simulink model "flightController"  (Simulink 9.1)
settings: Solver=ode3  StartTime=0  StopTime=TFinal  FixedStep=Ts  RelTol=1e-3  EnableMultiTasking=on
undefined symbols (not defined in the file): Controller, DiscIntNeverNeededParam, g, Ts, Vehicle
libraries: F_Line_block x89
settings Model: LogicAnalyzerSignalOrdering=201c873a-a194-43e1-85c1-7820e482cbc3,e6e4670c-19f9-4e85-8601-519539bde157  Creator=The MathWorks, Inc.  LastModifiedBy=dongw
settings DataIOCC: LimitDataPoints=on
settings OptimizationCC: BlockReduction=off  DefaultParameterBehavior=Inlined  BufferReuse=off  PassReuseOutputArgsThreshold=0  LifeSpan=auto
settings DebuggingCC: AlgebraicLoopMsg=none  UnderspecifiedInitializationDetection=Simplified  MergeDetectMultiDrivingBlocksExec=error  ParameterPrecisionLossMsg=none  ParameterTunabilityLossMsg=error  UnconnectedInputMsg=none  UnconnectedOutputMsg=none  UnconnectedLineMsg=none  BusObjectLabelMismatch=error
settings HardwareCC: ProdLargestAtomicInteger=Long  ProdLargestAtomicFloat=Float  ProdIntDivRoundTo=Zero  ProdEndianess=LittleEndian  ProdHWDeviceType=ARM Compatible->ARM 9
settings ModelReferenceCC: ModelReferenceNumInstancesAllowed=Single
settings RTWCC: GenerateReport=on  LaunchReport=on
settings CodeAppCC: ForceParamTrailComments=on  MaxIdLength=63  OperatorAnnotations=on  MATLABSourceComments=on
settings GRTTargetCC: CombineOutputUpdateFcns=on  GRTInterface=off
settings ConfigComp: CovSFcnEnable=off

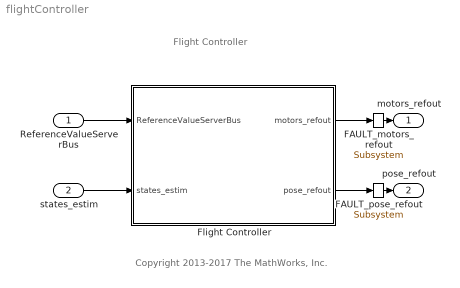
== system flightController ==
  note: Flight Controller
  note: Copyright 2013-2017 The MathWorks, Inc.
  ReferenceValueServerBus : Inport  OutDataTypeStr=Bus: CommandBus  BusOutputAsStruct=on
  states_estim : Inport  Port=2  OutDataTypeStr=Bus: statesEstim_t  BusOutputAsStruct=on
  Flight Controller : Subsystem
  motors_refout : Outport
  FAULT_motors_refout : F_Line_block/Subsystem
  pose_refout : Outport  Port=2
  FAULT_pose_refout : F_Line_block/Subsystem
  wires:
  ReferenceValueServerBus/1 -> Flight Controller/1(ReferenceValueServerBus)
  states_estim/1 -> Flight Controller/2(states_estim)
  Flight Controller/2(pose_refout) -> FAULT_pose_refout/1
  FAULT_pose_refout/1 -> pose_refout/1
  Flight Controller/1(motors_refout) -> FAULT_motors_refout/1
  FAULT_motors_refout/1 -> motors_refout/1

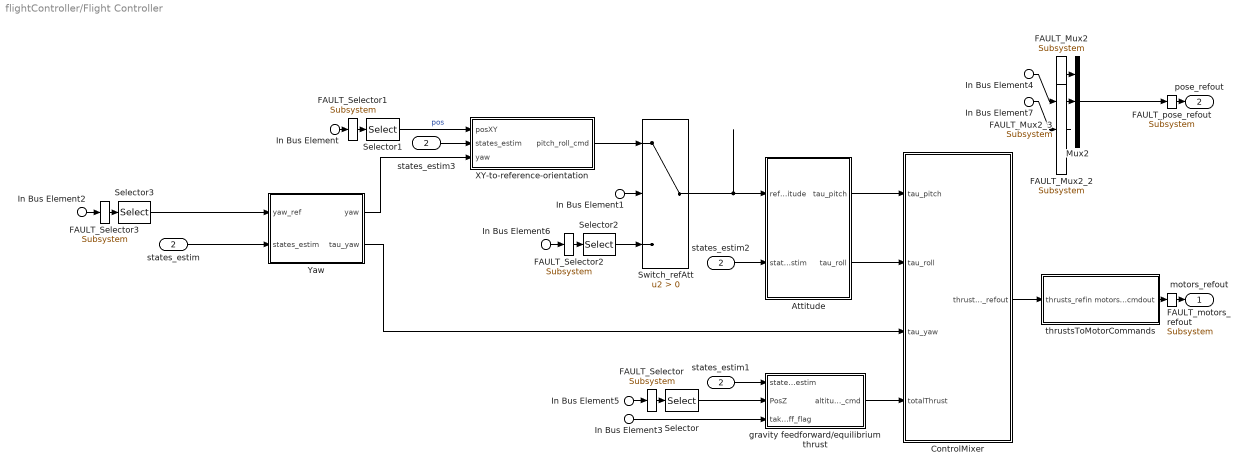
== system flightController/Flight Controller ==
  In Bus Element1 : Inport  PortName=ReferenceValueServerBus  Element=controlModePosVSOrient
  In Bus Element : Inport  PortName=ReferenceValueServerBus  Element=pos_ref
  In Bus Element4 : Inport  PortName=ReferenceValueServerBus  Element=pos_ref
  In Bus Element5 : Inport  PortName=ReferenceValueServerBus  Element=pos_ref
  In Bus Element2 : Inport  PortName=ReferenceValueServerBus  Element=orient_ref
  In Bus Element6 : Inport  PortName=ReferenceValueServerBus  Element=orient_ref
  In Bus Element7 : Inport  PortName=ReferenceValueServerBus  Element=orient_ref
  In Bus Element3 : Inport  PortName=ReferenceValueServerBus  Element=takeoff_flag
  states_estim : Inport  Port=2
  Attitude : Subsystem
  ControlMixer : Subsystem
  Mux2 : Mux  Inputs=3
  FAULT_Mux2 : F_Line_block/Subsystem
  FAULT_Mux2_2 : F_Line_block/Subsystem
  FAULT_Mux2_3 : F_Line_block/Subsystem
  Selector : Selector  InputPortWidth=3  IndexOptions=Index vector (dialog)  Indices=3  OutputSizes=1
  FAULT_Selector{,1..3} (4 alike) : F_Line_block/Subsystem
  Selector1 : Selector  InputPortWidth=3  IndexOptions=Index vector (dialog)  Indices=[1 2]  OutputSizes=1
  Selector2 : Selector  InputPortWidth=3  IndexOptions=Index vector (dialog)  Indices=[2 3]  OutputSizes=1
  Selector3 : Selector  InputPortWidth=3  IndexOptions=Index vector (dialog)  Indices=1  OutputSizes=1
  Switch_refAtt : Switch  Criteria=u2 > Threshold
  XY-to-reference-orientation : Subsystem
  Yaw : Subsystem
  gravity feedforward/equilibrium thrust : Subsystem
  states_estim1 : InportShadow  Port=2
  states_estim2 : InportShadow  Port=2
  states_estim3 : InportShadow  Port=2
  thrustsToMotorCommands : Subsystem
  motors_refout : Outport
  FAULT_motors_refout : F_Line_block/Subsystem
  pose_refout : Outport  Port=2
  FAULT_pose_refout : F_Line_block/Subsystem
  wires:
  thrustsToMotorCommands/1(motors_cmdout) -> FAULT_motors_refout/1
  FAULT_motors_refout/1 -> motors_refout/1
  In Bus Element1/1 -> Switch_refAtt/2
  XY-to-reference-orientation/1(pitch_roll_cmd) -> Switch_refAtt/1
  In Bus Element2/1 -> FAULT_Selector3/1
  FAULT_Selector3/1 -> Selector3/1
  In Bus Element/1 -> FAULT_Selector1/1
  FAULT_Selector1/1 -> Selector1/1
  Selector3/1 -> Yaw/1(yaw_ref)
  Selector1/1 -> XY-to-reference-orientation/1(posXY)  "pos"
  ControlMixer/1(thrusts_refout) -> thrustsToMotorCommands/1(thrusts_refin)
  In Bus Element3/1 -> gravity feedforward/equilibrium thrust/3(takeoff_flag)
  states_estim/1 -> Yaw/2(states_estim)
  Switch_refAtt/1 -> Attitude/1(refAttitude)
  ?FAULT_Sum4/1 -> ?Sum4/1
  FAULT_Mux2/1 -> Mux2/1
  Yaw/1(yaw) -> XY-to-reference-orientation/3(yaw)
  gravity feedforward/equilibrium thrust/1(altitude_cmd) -> ControlMixer/4(totalThrust)
  Mux2/1 -> FAULT_pose_refout/1
  FAULT_pose_refout/1 -> pose_refout/1
  Attitude/1(tau_pitch) -> ControlMixer/1(tau_pitch)
  Attitude/2(tau_roll) -> ControlMixer/2(tau_roll)
  Yaw/2(tau_yaw) -> ControlMixer/3(tau_yaw)
  states_estim1/1 -> gravity feedforward/equilibrium thrust/1(states_estim)
  states_estim2/1 -> Attitude/2(states_estim)
  states_estim3/1 -> XY-to-reference-orientation/2(states_estim)
  In Bus Element4/1 -> FAULT_Mux2/1
  FAULT_Mux2/1 -> Mux2/1
  Selector/1 -> gravity feedforward/equilibrium thrust/2(PosZ)
  In Bus Element5/1 -> FAULT_Selector/1
  FAULT_Selector/1 -> Selector/1
  In Bus Element6/1 -> FAULT_Selector2/1
  FAULT_Selector2/1 -> Selector2/1
  Selector2/1 -> Switch_refAtt/3
  In Bus Element7/1 -> FAULT_Mux2_2/1
  FAULT_Mux2_2/1 -> Mux2/2

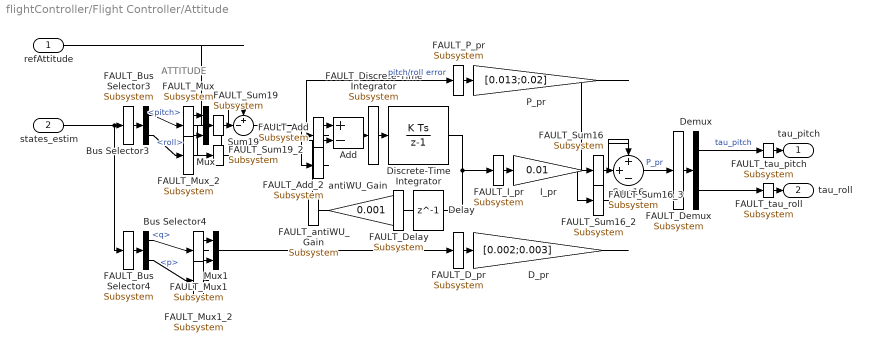
== system flightController/Flight Controller/Attitude ==
  note: ATTITUDE
  refAttitude : Inport
  states_estim : Inport  Port=2
  Add : Sum  Inputs=+-
  FAULT_Add : F_Line_block/Subsystem
  FAULT_Add_2 : F_Line_block/Subsystem
  Bus Selector3 : BusSelector  OutputSignals=pitch,roll
  FAULT_Bus Selector3 : F_Line_block/Subsystem
  Bus Selector4 : BusSelector  OutputSignals=q,p
  FAULT_Bus Selector4 : F_Line_block/Subsystem
  D_pr : Gain  Gain=[0.002;0.003]
  FAULT_D_pr : F_Line_block/Subsystem
  Delay : Delay  DelayLength=1  InitialCondition=0
  FAULT_Delay : F_Line_block/Subsystem
  Demux : Demux  Outputs=2
  FAULT_Demux : F_Line_block/Subsystem
  Discrete-Time Integrator : DiscreteIntegrator  SampleTime=Ts  LimitOutput=on  UpperSaturationLimit=2  LowerSaturationLimit=-2  ICPrevOutput=DiscIntNeverNeededParam  ICPrevScaledInput=DiscIntNeverNeededParam
  FAULT_Discrete-Time Integrator : F_Line_block/Subsystem
  I_pr : Gain  Gain=0.01
  FAULT_I_pr : F_Line_block/Subsystem
  Mux : Mux  Inputs=2
  FAULT_Mux : F_Line_block/Subsystem
  FAULT_Mux_2 : F_Line_block/Subsystem
  Mux1 : Mux  Inputs=2
  FAULT_Mux1 : F_Line_block/Subsystem
  FAULT_Mux1_2 : F_Line_block/Subsystem
  P_pr : Gain  Gain=[0.013;0.02]
  FAULT_P_pr : F_Line_block/Subsystem
  Sum16 : Sum  Inputs=++-  AccumDataTypeStr=single  OutDataTypeStr=single  SaturateOnIntegerOverflow=on
  FAULT_Sum16 : F_Line_block/Subsystem
  FAULT_Sum16_2 : F_Line_block/Subsystem
  FAULT_Sum16_3 : F_Line_block/Subsystem
  Sum19 : Sum  Inputs=+-|
  FAULT_Sum19 : F_Line_block/Subsystem
  FAULT_Sum19_2 : F_Line_block/Subsystem
  antiWU_Gain : Gain  Gain=0.001
  FAULT_antiWU_Gain : F_Line_block/Subsystem
  tau_pitch : Outport
  FAULT_tau_pitch : F_Line_block/Subsystem
  tau_roll : Outport  Port=2
  FAULT_tau_roll : F_Line_block/Subsystem
  wires:
  Sum16/1 -> FAULT_Demux/1  "P_pr"
  FAULT_Demux/1 -> Demux/1
  antiWU_Gain/1 -> FAULT_Add_2/1
  FAULT_Add_2/1 -> Add/2
  Add/1 -> FAULT_Discrete-Time Integrator/1
  FAULT_Discrete-Time Integrator/1 -> Discrete-Time Integrator/1
  Bus Selector3/1 -> FAULT_Mux/1  "<pitch>"
  FAULT_Mux/1 -> Mux/1
  Bus Selector4/1 -> FAULT_Mux1/1  "<q>"
  FAULT_Mux1/1 -> Mux1/1
  P_pr/1 -> FAULT_Sum16/1
  FAULT_Sum16/1 -> Sum16/1
  I_pr/1 -> FAULT_Sum16_2/1
  FAULT_Sum16_2/1 -> Sum16/2
  Sum19/1 -> FAULT_Add/1, FAULT_P_pr/1  "pitch/roll error"
  FAULT_Add/1 -> Add/1
  FAULT_P_pr/1 -> P_pr/1
  Discrete-Time Integrator/1 -> FAULT_Delay/1, FAULT_I_pr/1
  FAULT_Delay/1 -> Delay/1
  FAULT_I_pr/1 -> I_pr/1
  Delay/1 -> FAULT_antiWU_Gain/1
  FAULT_antiWU_Gain/1 -> antiWU_Gain/1
  Demux/1 -> FAULT_tau_pitch/1  "tau_pitch"
  FAULT_tau_pitch/1 -> tau_pitch/1
  Demux/2 -> FAULT_tau_roll/1
  FAULT_tau_roll/1 -> tau_roll/1
  D_pr/1 -> ?
  FAULT_Sum16/1 -> Sum16/1
  states_estim/1 -> FAULT_Bus Selector3/1, FAULT_Bus Selector4/1
  FAULT_Bus Selector3/1 -> Bus Selector3/1
  FAULT_Bus Selector4/1 -> Bus Selector4/1
  refAttitude/1 -> FAULT_Sum19/1
  FAULT_Sum19/1 -> Sum19/1
  Mux/1 -> FAULT_Sum19_2/1
  FAULT_Sum19_2/1 -> Sum19/2
  Bus Selector3/2 -> FAULT_Mux_2/1  "<roll>"
  FAULT_Mux_2/1 -> Mux/2
  Mux1/1 -> FAULT_D_pr/1
  FAULT_D_pr/1 -> D_pr/1
  Bus Selector4/2 -> FAULT_Mux1_2/1  "<p>"
  FAULT_Mux1_2/1 -> Mux1/2

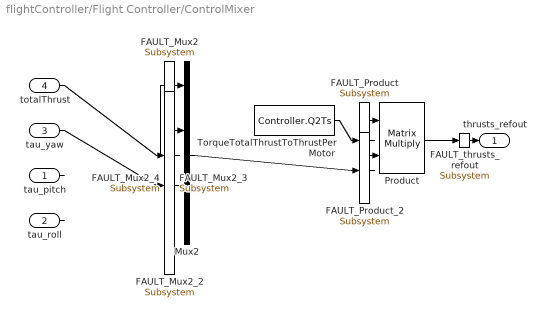
== system flightController/Flight Controller/ControlMixer ==
  tau_pitch : Inport
  tau_roll : Inport  Port=2
  tau_yaw : Inport  Port=3
  totalThrust : Inport  Port=4
  Mux2 : Mux
  FAULT_Mux2 : F_Line_block/Subsystem
  FAULT_Mux2_2 : F_Line_block/Subsystem
  FAULT_Mux2_3 : F_Line_block/Subsystem
  FAULT_Mux2_4 : F_Line_block/Subsystem
  Product : Product  Multiplication=Matrix(*)  RndMeth=Zero
  FAULT_Product : F_Line_block/Subsystem
  FAULT_Product_2 : F_Line_block/Subsystem
  TorqueTotalThrustToThrustPerMotor : Constant  Value=Controller.Q2Ts  OutDataTypeStr=single
  thrusts_refout : Outport
  FAULT_thrusts_refout : F_Line_block/Subsystem
  wires:
  Product/1 -> FAULT_thrusts_refout/1
  FAULT_thrusts_refout/1 -> thrusts_refout/1
  tau_roll/1 -> ?
  FAULT_Mux2/1 -> Mux2/1
  tau_pitch/1 -> ?
  FAULT_Mux2/1 -> Mux2/1
  tau_yaw/1 -> FAULT_Mux2_2/1
  FAULT_Mux2_2/1 -> Mux2/2
  totalThrust/1 -> FAULT_Mux2/1
  FAULT_Mux2/1 -> Mux2/1
  TorqueTotalThrustToThrustPerMotor/1 -> FAULT_Product/1
  FAULT_Product/1 -> Product/1
  Mux2/1 -> FAULT_Product_2/1
  FAULT_Product_2/1 -> Product/2

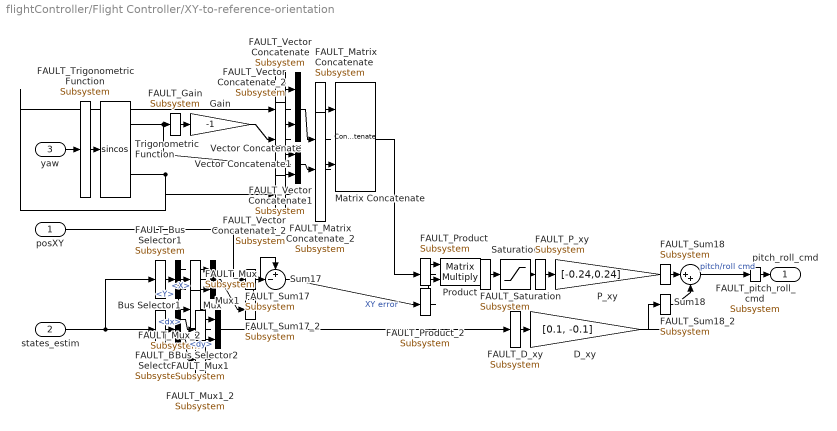
== system flightController/Flight Controller/XY-to-reference-orientation ==
  posXY : Inport
  states_estim : Inport  Port=2
  yaw : Inport  Port=3
  Bus Selector1 : BusSelector  OutputSignals=X,Y
  FAULT_Bus Selector1 : F_Line_block/Subsystem
  Bus Selector2 : BusSelector  OutputSignals=dx,dy
  FAULT_Bus Selector2 : F_Line_block/Subsystem
  D_xy : Gain  Gain=[0.1, -0.1]  ParamDataTypeStr=single  OutDataTypeStr=single  SaturateOnIntegerOverflow=on
  FAULT_D_xy : F_Line_block/Subsystem
  Gain : Gain  Gain=-1
  FAULT_Gain : F_Line_block/Subsystem
  Matrix Concatenate : Concatenate  Mode=Multidimensional array  ConcatenateDimension=2
  FAULT_Matrix Concatenate : F_Line_block/Subsystem
  FAULT_Matrix Concatenate_2 : F_Line_block/Subsystem
  Mux : Mux  Inputs=2
  FAULT_Mux : F_Line_block/Subsystem
  FAULT_Mux_2 : F_Line_block/Subsystem
  Mux1 : Mux  Inputs=2
  FAULT_Mux1 : F_Line_block/Subsystem
  FAULT_Mux1_2 : F_Line_block/Subsystem
  P_xy : Gain  Gain=[-0.24,0.24]  ParamDataTypeStr=single  OutDataTypeStr=single  SaturateOnIntegerOverflow=on
  FAULT_P_xy : F_Line_block/Subsystem
  Product : Product  Multiplication=Matrix(*)  OutDataTypeStr=single  RndMeth=Zero
  FAULT_Product : F_Line_block/Subsystem
  FAULT_Product_2 : F_Line_block/Subsystem
  Saturation : Saturate  UpperLimit=3  LowerLimit=-3  OutDataTypeStr=single
  FAULT_Saturation : F_Line_block/Subsystem
  Sum17 : Sum  Inputs=+-|  AccumDataTypeStr=single
  FAULT_Sum17 : F_Line_block/Subsystem
  FAULT_Sum17_2 : F_Line_block/Subsystem
  Sum18 : Sum  Inputs=|++  AccumDataTypeStr=single  OutDataTypeStr=single  SaturateOnIntegerOverflow=on
  FAULT_Sum18 : F_Line_block/Subsystem
  FAULT_Sum18_2 : F_Line_block/Subsystem
  Trigonometric Function : Trigonometry  Operator=sincos
  FAULT_Trigonometric Function : F_Line_block/Subsystem
  Vector Concatenate : Concatenate
  FAULT_Vector Concatenate : F_Line_block/Subsystem
  FAULT_Vector Concatenate_2 : F_Line_block/Subsystem
  Vector Concatenate1 : Concatenate
  FAULT_Vector Concatenate1 : F_Line_block/Subsystem
  FAULT_Vector Concatenate1_2 : F_Line_block/Subsystem
  pitch_roll_cmd : Outport
  FAULT_pitch_roll_cmd : F_Line_block/Subsystem
  wires:
  yaw/1 -> FAULT_Trigonometric Function/1
  FAULT_Trigonometric Function/1 -> Trigonometric Function/1
  Saturation/1 -> FAULT_P_xy/1
  FAULT_P_xy/1 -> P_xy/1
  P_xy/1 -> FAULT_Sum18/1
  FAULT_Sum18/1 -> Sum18/1
  Sum17/1 -> FAULT_Product_2/1  "XY error"
  FAULT_Product_2/1 -> Product/2
  posXY/1 -> FAULT_Sum17/1
  FAULT_Sum17/1 -> Sum17/1
  Bus Selector2/1 -> FAULT_Mux1/1  "<dx>"
  FAULT_Mux1/1 -> Mux1/1
  states_estim/1 -> FAULT_Bus Selector1/1, FAULT_Bus Selector2/1
  FAULT_Bus Selector1/1 -> Bus Selector1/1
  FAULT_Bus Selector2/1 -> Bus Selector2/1
  Sum18/1 -> FAULT_pitch_roll_cmd/1  "pitch/roll cmd"
  FAULT_pitch_roll_cmd/1 -> pitch_roll_cmd/1
  D_xy/1 -> FAULT_Sum18_2/1
  FAULT_Sum18_2/1 -> Sum18/2
  Bus Selector1/1 -> FAULT_Mux/1  "<X>"
  FAULT_Mux/1 -> Mux/1
  Product/1 -> FAULT_Saturation/1
  FAULT_Saturation/1 -> Saturation/1
  Trigonometric Function/1 -> FAULT_Gain/1, FAULT_Vector Concatenate1/1
  FAULT_Gain/1 -> Gain/1
  FAULT_Vector Concatenate1/1 -> Vector Concatenate1/1
  Trigonometric Function/2 -> FAULT_Vector Concatenate1_2/1, FAULT_Vector Concatenate/1
  FAULT_Vector Concatenate1_2/1 -> Vector Concatenate1/2
  FAULT_Vector Concatenate/1 -> Vector Concatenate/1
  Gain/1 -> FAULT_Vector Concatenate_2/1
  FAULT_Vector Concatenate_2/1 -> Vector Concatenate/2
  Vector Concatenate/1 -> FAULT_Matrix Concatenate/1
  FAULT_Matrix Concatenate/1 -> Matrix Concatenate/1
  Vector Concatenate1/1 -> FAULT_Matrix Concatenate_2/1
  FAULT_Matrix Concatenate_2/1 -> Matrix Concatenate/2
  Matrix Concatenate/1 -> FAULT_Product/1
  FAULT_Product/1 -> Product/1
  Bus Selector1/2 -> FAULT_Mux_2/1  "<Y>"
  FAULT_Mux_2/1 -> Mux/2
  Mux/1 -> FAULT_Sum17_2/1
  FAULT_Sum17_2/1 -> Sum17/2
  Mux1/1 -> FAULT_D_xy/1
  FAULT_D_xy/1 -> D_xy/1
  Bus Selector2/2 -> FAULT_Mux1_2/1  "<dy>"
  FAULT_Mux1_2/1 -> Mux1/2

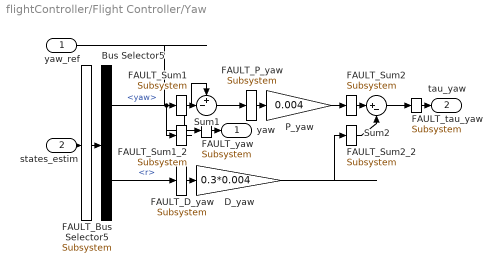
== system flightController/Flight Controller/Yaw ==
  yaw_ref : Inport
  states_estim : Inport  Port=2
  Bus Selector5 : BusSelector  OutputSignals=yaw,r
  FAULT_Bus Selector5 : F_Line_block/Subsystem
  D_yaw : Gain  Gain=0.3*0.004
  FAULT_D_yaw : F_Line_block/Subsystem
  P_yaw : Gain  Gain=0.004  ParamDataTypeStr=single  OutDataTypeStr=single
  FAULT_P_yaw : F_Line_block/Subsystem
  Sum1 : Sum  Inputs=+-|  AccumDataTypeStr=single  OutDataTypeStr=single  SaturateOnIntegerOverflow=on
  FAULT_Sum1 : F_Line_block/Subsystem
  FAULT_Sum1_2 : F_Line_block/Subsystem
  Sum2 : Sum  Inputs=|+-
  FAULT_Sum2 : F_Line_block/Subsystem
  FAULT_Sum2_2 : F_Line_block/Subsystem
  yaw : Outport
  FAULT_yaw : F_Line_block/Subsystem
  tau_yaw : Outport  Port=2
  FAULT_tau_yaw : F_Line_block/Subsystem
  wires:
  D_yaw/1 -> FAULT_Sum2_2/1
  FAULT_Sum2_2/1 -> Sum2/2
  P_yaw/1 -> FAULT_Sum2/1
  FAULT_Sum2/1 -> Sum2/1
  Bus Selector5/2 -> FAULT_D_yaw/1  "<r>"
  FAULT_D_yaw/1 -> D_yaw/1
  Sum1/1 -> FAULT_P_yaw/1
  FAULT_P_yaw/1 -> P_yaw/1
  states_estim/1 -> FAULT_Bus Selector5/1
  FAULT_Bus Selector5/1 -> Bus Selector5/1
  Sum2/1 -> FAULT_tau_yaw/1
  FAULT_tau_yaw/1 -> tau_yaw/1
  Bus Selector5/1 -> FAULT_yaw/1, FAULT_Sum1_2/1  "<yaw>"
  FAULT_yaw/1 -> yaw/1
  FAULT_Sum1_2/1 -> Sum1/2
  yaw_ref/1 -> FAULT_Sum1/1
  FAULT_Sum1/1 -> Sum1/1

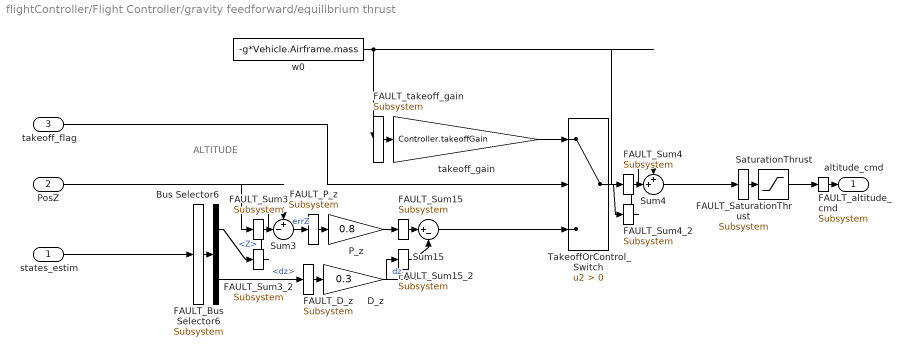
== system flightController/Flight Controller/gravity feedforward/equilibrium thrust ==
  note: ALTITUDE
  states_estim : Inport
  PosZ : Inport  Port=2
  takeoff_flag : Inport  Port=3
  Bus Selector6 : BusSelector  OutputSignals=Z,dz
  FAULT_Bus Selector6 : F_Line_block/Subsystem
  D_z : Gain  Gain=0.3  ParamDataTypeStr=single  OutDataTypeStr=single  SaturateOnIntegerOverflow=on
  FAULT_D_z : F_Line_block/Subsystem
  P_z : Gain  Gain=0.8  ParamDataTypeStr=single  OutDataTypeStr=single  SaturateOnIntegerOverflow=on
  FAULT_P_z : F_Line_block/Subsystem
  SaturationThrust : Saturate  UpperLimit=4*Controller.totalThrustMaxRelative*Controller.motorsThrustPerMotorMax  LowerLimit=-4*Controller.totalThrustMaxRelative*Controller.motorsThrustPerMotorMax  OutDataTypeStr=single
  FAULT_SaturationThrust : F_Line_block/Subsystem
  Sum15 : Sum  Inputs=|+-  AccumDataTypeStr=single  OutDataTypeStr=single  SaturateOnIntegerOverflow=on
  FAULT_Sum15 : F_Line_block/Subsystem
  FAULT_Sum15_2 : F_Line_block/Subsystem
  Sum3 : Sum  Inputs=+-|  AccumDataTypeStr=single  OutDataTypeStr=single  SaturateOnIntegerOverflow=on
  FAULT_Sum3 : F_Line_block/Subsystem
  FAULT_Sum3_2 : F_Line_block/Subsystem
  Sum4 : Sum  Inputs=++|  AccumDataTypeStr=single  OutDataTypeStr=single  SaturateOnIntegerOverflow=on
  FAULT_Sum4 : F_Line_block/Subsystem
  FAULT_Sum4_2 : F_Line_block/Subsystem
  TakeoffOrControl_Switch : Switch  Criteria=u2 > Threshold
  takeoff_gain : Gain  Gain=Controller.takeoffGain  ParamDataTypeStr=single  OutDataTypeStr=single  SaturateOnIntegerOverflow=on
  FAULT_takeoff_gain : F_Line_block/Subsystem
  w0 : Constant  Value=-g*Vehicle.Airframe.mass  OutDataTypeStr=single  SampleTime=Ts
  altitude_cmd : Outport
  FAULT_altitude_cmd : F_Line_block/Subsystem
  wires:
  Sum3/1 -> FAULT_P_z/1  "errZ"
  FAULT_P_z/1 -> P_z/1
  TakeoffOrControl_Switch/1 -> FAULT_Sum4_2/1
  FAULT_Sum4_2/1 -> Sum4/2
  Bus Selector6/1 -> FAULT_Sum3_2/1  "<Z>"
  FAULT_Sum3_2/1 -> Sum3/2
  Bus Selector6/2 -> FAULT_D_z/1  "<dz>"
  FAULT_D_z/1 -> D_z/1
  w0/1 -> FAULT_Sum4/1, FAULT_takeoff_gain/1
  FAULT_Sum4/1 -> Sum4/1
  FAULT_takeoff_gain/1 -> takeoff_gain/1
  D_z/1 -> FAULT_Sum15_2/1  "dz"
  FAULT_Sum15_2/1 -> Sum15/2
  takeoff_gain/1 -> TakeoffOrControl_Switch/1
  takeoff_flag/1 -> TakeoffOrControl_Switch/2
  PosZ/1 -> FAULT_Sum3/1
  FAULT_Sum3/1 -> Sum3/1
  P_z/1 -> FAULT_Sum15/1
  FAULT_Sum15/1 -> Sum15/1
  Sum15/1 -> TakeoffOrControl_Switch/3
  Sum4/1 -> FAULT_SaturationThrust/1
  FAULT_SaturationThrust/1 -> SaturationThrust/1
  SaturationThrust/1 -> FAULT_altitude_cmd/1
  FAULT_altitude_cmd/1 -> altitude_cmd/1
  states_estim/1 -> FAULT_Bus Selector6/1
  FAULT_Bus Selector6/1 -> Bus Selector6/1

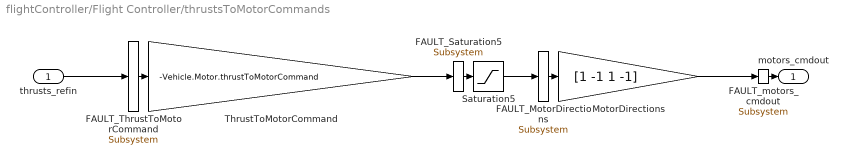
== system flightController/Flight Controller/thrustsToMotorCommands ==
  thrusts_refin : Inport
  MotorDirections : Gain  Gain=[1 -1 1 -1]
  FAULT_MotorDirections : F_Line_block/Subsystem
  Saturation5 : Saturate  UpperLimit=Vehicle.Motor.maxLimit  LowerLimit=Vehicle.Motor.minLimit
  FAULT_Saturation5 : F_Line_block/Subsystem
  ThrustToMotorCommand : Gain  Gain=-Vehicle.Motor.thrustToMotorCommand
  FAULT_ThrustToMotorCommand : F_Line_block/Subsystem
  motors_cmdout : Outport
  FAULT_motors_cmdout : F_Line_block/Subsystem
  wires:
  Saturation5/1 -> FAULT_MotorDirections/1
  FAULT_MotorDirections/1 -> MotorDirections/1
  MotorDirections/1 -> FAULT_motors_cmdout/1
  FAULT_motors_cmdout/1 -> motors_cmdout/1
  ThrustToMotorCommand/1 -> FAULT_Saturation5/1
  FAULT_Saturation5/1 -> Saturation5/1
  thrusts_refin/1 -> FAULT_ThrustToMotorCommand/1
  FAULT_ThrustToMotorCommand/1 -> ThrustToMotorCommand/1
